simulink model "quadcoptermodel2"  (R2015a)
settings: Solver=ode45  StartTime=0.0  StopTime=10.0  RelTol=1e-3
values from neighbouring files (symbols this model uses):
  A = [ 0 0 0 1 0 0 0 0 ... (first row only)    [update_state_matrices.m]
  B = [   0 0 0 0 ... (first row only)    [update_state_matrices.m]
  C = eye(8)    [update_state_matrices.m]
  D = zeros(8,4)    [update_state_matrices.m]
settings Model: CovSFcnEnable=off  Creator=Mikael  LastModifiedBy=bjornni
settings DebuggingCC: SolverPrmCheckMsg=warning

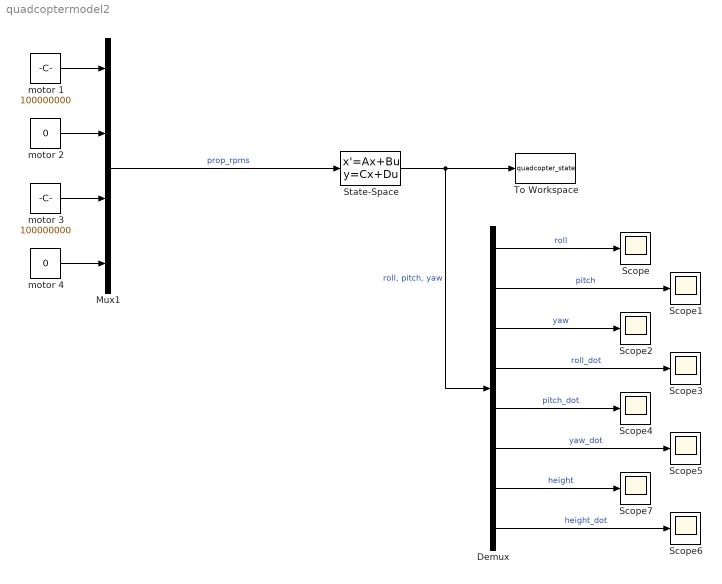
== system quadcoptermodel2 ==
  Demux : Demux  Outputs=8
  Mux1 : Mux
  Scope{,1..7} (8 alike) : Scope
      Scope2 settings: SaveName=ScopeData2
      Scope3 settings: SaveName=ScopeData3
      Scope4 settings: SaveName=ScopeData4
      Scope5 settings: SaveName=ScopeData5
      Scope6 settings: SaveName=ScopeData6
      Scope7 settings: SaveName=ScopeData7
  State-Space : StateSpace  A=A  B=B  C=C  D=D  X0=0
  To Workspace : ToWorkspace  VariableName=quadcopter_state  SaveFormat=Structure With Time  SampleTime=-1
  motor 1 : Constant  Value=100000000
  motor 2 : Constant  Value=0
  motor 3 : Constant  Value=100000000
  motor 4 : Constant  Value=0
  wires:
  motor 1/1 -> Mux1/1
  motor 2/1 -> Mux1/2
  motor 3/1 -> Mux1/3
  motor 4/1 -> Mux1/4
  State-Space/1 -> Demux/1, To Workspace/1  "roll, pitch, yaw"
  Mux1/1 -> State-Space/1  "prop_rpms"
  Demux/8 -> Scope6/1  "height_dot"
  Demux/1 -> Scope/1  "roll"
  Demux/2 -> Scope1/1  "pitch"
  Demux/3 -> Scope2/1  "yaw"
  Demux/4 -> Scope3/1  "roll_dot"
  Demux/5 -> Scope4/1  "pitch_dot"
  Demux/6 -> Scope5/1  "yaw_dot"
  Demux/7 -> Scope7/1  "height"
